simulink model "Telemetry_Test_Airshow"  (Simulink 8.0)
settings: Solver=ode5  StartTime=0.0  StopTime=inf  FixedStep=sample_time_Vicon  RelTol=1e-3
InitFcn:
  | sample_time_Vicon = 0.004;
  | sample_time=0.02;
  | DeltaT = sample_time;
  | H0 = -0.36;
  | Kl = 1;
  | Omega_r =1.1; %1.3
settings Model: Creator=ttcl3  LastModifiedBy=CHIEW
settings SolverCC: MaxConsecutiveMinStep=auto
settings DataIOCC: SignalLoggingSaveFormat=ModelDataLogs
settings OptimizationCC: EfficientMapNaN2IntZero=off
settings DebuggingCC: MultiTaskRateTransMsg=warning  FcnCallInpInsideContextMsg=UseLocalSettings
settings HardwareCC: TargetIntDivRoundTo=Zero  TargetEndianess=LittleEndian  TargetHWDeviceType=MATLAB Host  ProdEqTarget=off
settings SFSimCC: SimParseCustomCode=off
settings CodeAppCC: MaxIdLength=128
settings GRTTargetCC: CombineOutputUpdateFcns=off  GRTInterface=on

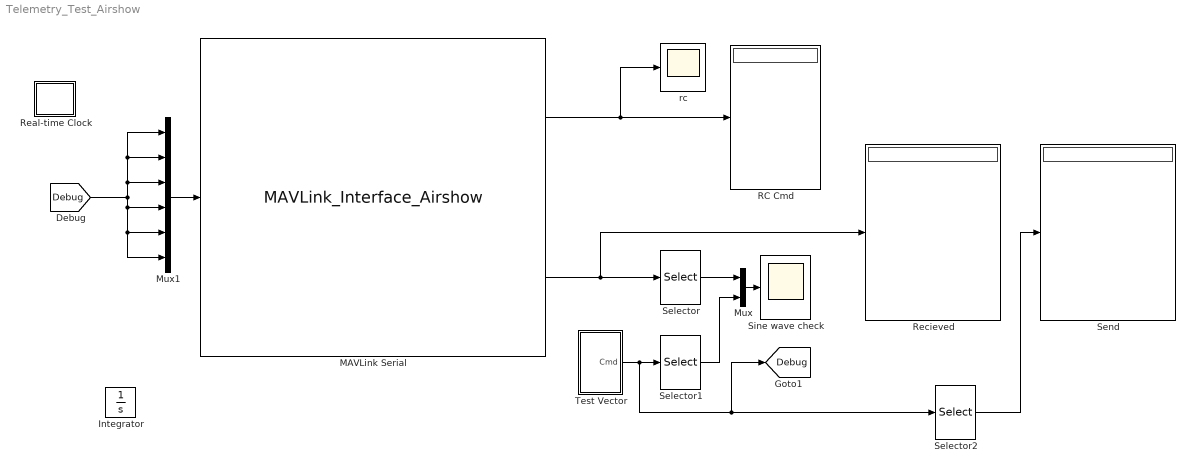
== system Telemetry_Test_Airshow ==
  Integrator : Integrator
  MAVLink Serial : S-Function  FunctionName=MAVLink_Interface_Airshow  Parameters=COM_Port,Baud_Rate,MSG_INPUT,MSG_OUTPUT  EnableBusSupport=off  mask{COM_Port='COM9', Baud_Rate=57600, ATTITUDE_OUT=on, RC_SCALED=on, Quads_1=off, Quads_2=off, Quads_3=off, Quads_4=off, Quads_5=off, Quads_6=on}
      mask prompts: COM_Port "COM Port"; Baud_Rate "Baud Rate"; ATTITUDE_OUT "DEBUG"; RC_SCALED "RC CHANNELS SCALED"; Quads_1 "1 Quad"; Quads_2 "2 Quad"; Quads_3 "3 Quad"; Quads_4 "4 Quad"; Quads_5 "5 Quad"; Quads_6 "6 Quad"
      mask init:
      | MSG_ID_NUM_INPUT = [ uint8(221) uint8(222) uint8(223) uint8(224) uint8(225) uint8(226)];
      | MSG_ID_NAME_INPUT = [Quads_1 Quads_2 Quads_3 Quads_4 Quads_5 Quads_6];
      | 
      | MSG_ID_NUM_OUTPUT = [uint8(34) uint8(30)];
      | MSG_ID_NAME_OUTPUT = [RC_SCALED ATTITUDE_OUT ];
      | 
      | idx_input = find(MSG_ID_NAME_INPUT);
      | MSG_INPUT = MSG_ID_NUM_INPUT(idx_input);
      | 
      | idx_output = find(MSG_ID_NAME_OUTPUT);
      | MSG_OUTPUT = MSG_ID_NUM_OUTPUT(idx_output);
      mask Display:
      | % Block image
      | image(imread('10-inch Quad Heat Map.png'));
      | 
      | %Label block
      | fprintf('MAVLink Serial\n%s\n%dbps', COM_Port,  Baud_Rate)
      | 
      | 
      | %Label input ports
      | 
      | in = 1;
      | if (Quads_1 == 1)
      |     port_label('input', in, 'Quads_1');
      |     in = in + 1;
      | end
      | 
      | if (Quads_2 == 1)
      |     port_label('input', in, 'Quads_2');
      |     in = in + 1;
      | end
      | 
      | if (Quads_3 == 1)
      |     port_label('input', in, 'Quads_3');
      |     in = in + 1;
      | end
      | 
      | if (Quads_4 == 1)
      |     port_label('input', in, 'Quads_4');
      |     in = in + 1;
      | end
      | 
      | if (Quads_5 == 1)
      |     port_label('input', in, 'Quads_5');
      |     in = in + 1;
      | end
      | 
      | 
      | if (Quads_6 == 1)
      |     port_label('input', in, 'Quads_6');
      |     in = in + 1;
      | end
      | %Label output ports
      | 
      | out = 1;
      | if (RC_SCALED == 1)
      |     port_label('output', out, 'RC CMD');
      |     out = out + 1;
      | end
      | 
      | if (ATTITUDE_OUT == 1)
      |     port_label('output', out, 'DEBUG');
      |     out = out + 1;
      | end
  Mux : Mux  Inputs=2
  Mux1 : Mux  Inputs=6
  RC Cmd : Display
  Real-time Clock : Subsystem  mask(Real-time Clock){sample_time=sample_time, tolerance=0.03}
      mask prompts: sample_time "Synchronize with real-time every n seconds:"; tolerance "Real-time warning tolerance (seconds):"
      mask help: Real-time Synchronization Block
      mask Help: This block synchronizes simulation time with the PC real-time clock or UNIX system clock. The first dialog entry is the period at which the clock is checked to insure real-time synchronization. The second dialog entry is the number of seconds that the simulation time must be within real-time before a warning is printed.
      mask Display: plot(0,0,100,100,[40,60,60,54,54,64,69,76,82,77,81,83,83,81,78,74,70,64,57,49,41,35,32,30,30,31,34,40,47,47,40,40],[90,90,85,85,80,79,76,87,80,70,64,57,49,41,33,28,24,22,21,23,25,31,37,46,56,65,73,78,80,85,85,90],[69,53,53],[64,50,73])
  Recieved : Display
  Selector : Selector  InputPortWidth=6  IndexOptions=Index vector (dialog)  Indices=[3]  OutputSizes=1
  Selector1 : Selector  InputPortWidth=6  IndexOptions=Index vector (dialog)  Indices=1  OutputSizes=1
  Selector2 : Selector  InputPortWidth=6  IndexOptions=Index vector (dialog)  Indices=[5 6 1 2 3 4]  OutputSizes=1
  Send : Display
  Sine wave check : Scope
      settings: TimeRange=10  YMin=-1  YMax=1  SaveName=ScopeData2
  Test Vector : Subsystem
  rc : Scope
      settings: TimeRange=10  YMin=-1  YMax=0.05
  tag scope: Debug=global
  wires:
  MAVLink Serial/1 -> RC Cmd/1, rc/1
  Mux/1 -> Sine wave check/1
  Selector/1 -> Mux/1
  Selector1/1 -> Mux/2
  MAVLink Serial/2 -> Recieved/1, Selector/1
  Test Vector/1(Cmd) -> [Debug], Selector2/1, Selector1/1
  Mux1/1 -> MAVLink Serial/1
  [Debug] -> Mux1/4, Mux1/5, Mux1/6, Mux1/1, Mux1/2, Mux1/3
  Selector2/1 -> Send/1

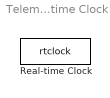
== system Telemetry_Test_Airshow/Real-time Clock ==
  Real-time Clock : S-Function  FunctionName=rtclock  Parameters=sample_time, tolerance  EnableBusSupport=off

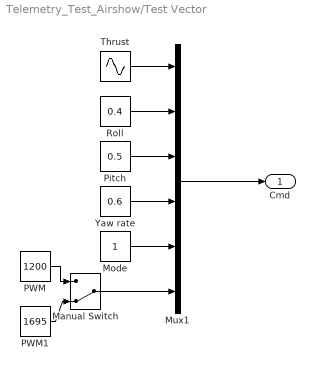
== system Telemetry_Test_Airshow/Test Vector ==
  Manual Switch : ManualSwitch  CurrentSetting=0
  Mode : Constant
  Mux1 : Mux  Inputs=6
  PWM : Constant  Value=1200
  PWM1 : Constant  Value=1695
  Pitch : Constant  Value=0.5
  Roll : Constant  Value=0.4
  Thrust : Sin  SampleTime=0
  Yaw rate : Constant  Value=0.6
  Cmd : Outport
  wires:
  Mode/1 -> Mux1/5
  Manual Switch/1 -> Mux1/6
  PWM/1 -> Manual Switch/1
  Thrust/1 -> Mux1/1
  Mux1/1 -> Cmd/1
  Roll/1 -> Mux1/2
  Pitch/1 -> Mux1/3
  Yaw rate/1 -> Mux1/4
  PWM1/1 -> Manual Switch/2
